simulink model "fen_control"  (Simulink 7.9)
settings: Solver=ode45  StartTime=0.0  StopTime=sim_stop_time  RelTol=1e-3
undefined symbols (not defined in the file): Ad, Bd, Cd_control, Dd_control, K_control, Ts, x_0
settings Model: Creator=matias  LastModifiedBy=matias
settings DebuggingCC: SolverPrmCheckMsg=none

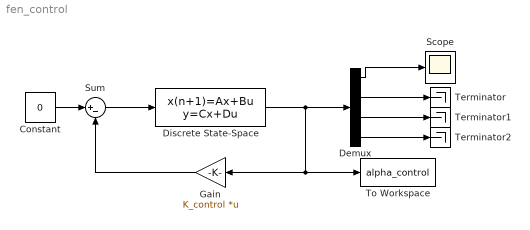
== system fen_control ==
  Constant : Constant  Value=0
  Demux : Demux
  Discrete State-Space : DiscreteStateSpace  A=Ad  B=Bd  C=Cd_control  D=Dd_control  X0=x_0  SampleTime=Ts
  Gain : Gain  Gain=K_control  Multiplication=Matrix(K*u)
  Scope : Scope
      settings: SaveName=control_alpha
  Sum : Sum  Inputs=|+-
  Terminator : Terminator
  Terminator1 : Terminator
  Terminator2 : Terminator
  To Workspace : ToWorkspace  VariableName=alpha_control  SampleTime=-1  SaveFormat=Timeseries
  wires:
  Discrete State-Space/1 -> Demux/1, Gain/1, To Workspace/1
  Constant/1 -> Sum/1
  Gain/1 -> Sum/2
  Sum/1 -> Discrete State-Space/1
  Demux/1 -> Scope/1
  Demux/2 -> Terminator/1
  Demux/3 -> Terminator1/1
  Demux/4 -> Terminator2/1
